simulink model "elevateur_L_BF"  (R2015b)
settings: Solver=ode45  StartTime=0.0  StopTime=10.0  RelTol=1e-3
undefined symbols (not defined in the file): A, B, C, D, Kd, Ki, Kp
settings Model: Creator=Administrator  LastModifiedBy=dsaussie
settings DataIOCC: SaveFormat=Array
settings DebuggingCC: UnderspecifiedInitializationDetection=Classic  MergeDetectMultiDrivingBlocksExec=none  SolverPrmCheckMsg=warning
settings HardwareCC: ProdBitPerPointer=32  ProdLargestAtomicFloat=None  ProdIntDivRoundTo=Undefined  ProdEndianess=Unspecified  ProdWordSize=32  ProdHWDeviceType=32-bit Generic
settings GRTTargetCC: GeneratePreprocessorConditionals=Disable all
settings ConfigComp: CovModelRefEnable=Off

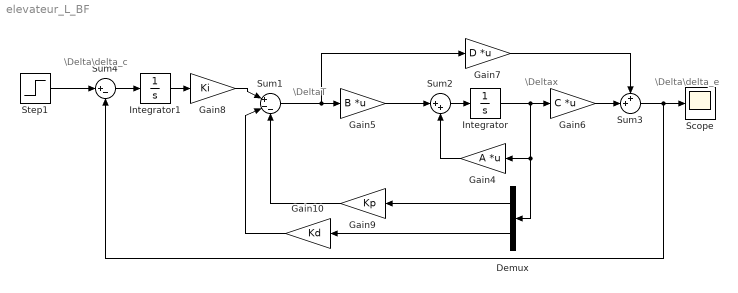
== system elevateur_L_BF ==
  note: \DeltaT
  note: \Deltax
  note: \Delta\delta_e
  note: \Delta\delta_c
  Demux : Demux  Outputs=2
  Gain10 : Gain  Gain=Kd
  Gain4 : Gain  Gain=A  Multiplication=Matrix(K*u)
  Gain5 : Gain  Gain=B  Multiplication=Matrix(K*u)
  Gain6 : Gain  Gain=C  Multiplication=Matrix(K*u)
  Gain7 : Gain  Gain=D  Multiplication=Matrix(K*u)
  Gain8 : Gain  Gain=Ki
  Gain9 : Gain  Gain=Kp
  Integrator : Integrator
  Integrator1 : Integrator
  Scope : Scope
  Step1 : Step  Time=0  SampleTime=0
  Sum1 : Sum  Inputs=|+--
  Sum2 : Sum  Inputs=|++
  Sum3 : Sum  Inputs=++|
  Sum4 : Sum  Inputs=|+-
  wires:
  Sum2/1 -> Integrator/1
  Integrator/1 -> Gain6/1, Demux/1, Gain4/1
  Gain4/1 -> Sum2/2
  Gain5/1 -> Sum2/1
  Sum1/1 -> Gain7/1, Gain5/1
  Gain6/1 -> Sum3/2
  Gain7/1 -> Sum3/1
  Step1/1 -> Sum4/1
  Sum3/1 -> Sum4/2, Scope/1
  Demux/1 -> Gain9/1
  Demux/2 -> Gain10/1
  Gain10/1 -> Sum1/2
  Gain9/1 -> Sum1/3
  Gain8/1 -> Sum1/1
  Integrator1/1 -> Gain8/1
  Sum4/1 -> Integrator1/1
